simulink library "dspbuff3"  (Simulink 5.0)
libraries: dspbuff3 x1
settings Model: RequirementInfo=9  CovMetricSettings=d  Creator=szlotkin  LastModifiedBy=mkhan  TargetHWChar=2  TargetHWWordLengths=8,16,32,32

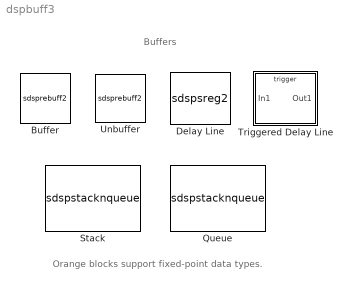
== system dspbuff3 ==
  note: Buffers
  note: Orange blocks support fixed-point data types.
  Buffer : S-Function  FunctionName=sdsprebuff2  Parameters=N,V,ic  mask(Buffer){N=64, V=0, ic=0}
      mask prompts: N "Output buffer size (per channel):"; V "Buffer overlap:"; ic "Initial conditions:"
      mask help:
      | Convert scalar samples to a frame output at a lower sample rate.  You can also convert a frame to a smaller or larger size with optional overlap.
      | For calculation of sample delay, see the rebuffer_delay function.
      mask init:
      | [x,y] = dspblkbuff('icon');
      settings: CopyFcn=dspfixptcopycallback
      mask Help: web(dspbhelp);
      mask Display: plot(x,y)
  Delay Line : S-Function  FunctionName=sdspsreg2  Parameters=siz,ic,directfeed  mask(Delay Line){siz=64, ic=0, directfeed=off}
      mask prompts: siz "Delay line size:"; ic "Initial conditions:"; directfeed "Allow directfeedthrough"
      mask help: Shift out delay line contents and store input data into start of delay line.
      settings: CopyFcn=dspfixptcopycallback
      mask Help: web(dspbhelp);
      mask Display: disp('Delay\nLine');
  Queue : S-Function  FunctionName=sdspstacknqueue  Parameters=trigger,depth,overflow,pes,eso,fso,nso,clr,clrOutport,1  mask(Queue){depth=8, trigger=Rising edge, overflow=Dynamic reallocation, pes=Warning, eso=off, fso=off, nso=off, clr=off, clrOutport=off}
      mask prompts: depth "Register size:"; trigger "Trigger type:"; overflow "Push onto full register:"; pes "Pop empty register:"; eso "Empty register output"; fso "Full register output"; nso "Output number of register entries"; clr "Clear input"; clrOutport "Clear output port on reset"
      mask help: Implements a queue, or "First In, First Out" (FIFO) register.
      mask init:
      | [si,so] = dspblkstack('icon', clr,eso,fso,nso);
      settings: CopyFcn=dspfixptcopycallback
      mask Help: web(dspbhelp);
      mask StyleString: edit,popup(Rising edge|Falling edge|Either edge|Non-zero sample),popup(Dynamic reallocation|Ignore|Warning|Error),popup(Ignore|Warning|Error),checkbox,checkbox,checkbox,checkbox,checkbox
      mask Display:
      | disp('Queue');
      | 
      | port_label('input',si(1).port, si(1).txt);
      | port_label('input',si(2).port, si(2).txt);
      | port_label('input',si(3).port, si(3).txt);
      | port_label('input',si(4).port, si(4).txt);
      | 
      | port_label('output',so(1).port, so(1).txt);
      | port_label('output',so(2).port, so(2).txt);
      | port_label('output',so(3).port, so(3).txt);
      | port_label('output',so(4).port, so(4).txt);
  Stack : S-Function  FunctionName=sdspstacknqueue  Parameters=trigger,depth,overflow,pes,eso,fso,nso,clr,clrOutport,0  mask(Stack){depth=8, trigger=Rising edge, overflow=Dynamic reallocation, pes=Warning, eso=off, fso=off, nso=off, clr=off, clrOutport=off}
      mask prompts: depth "Stack depth:"; trigger "Trigger type:"; overflow "Push full stack:"; pes "Pop empty stack:"; eso "Empty stack output"; fso "Full stack output"; nso "Output number of stack entries"; clr "Clear input"; clrOutport "Clear output port on reset"
      mask help: Implements a stack, or "Last In, First Out" (LIFO) register.
      mask init:
      | [si,so] = dspblkstack('icon', clr,eso,fso,nso);
      settings: CopyFcn=dspfixptcopycallback
      mask Help: web(dspbhelp);
      mask StyleString: edit,popup(Rising edge|Falling edge|Either edge|Non-zero sample),popup(Dynamic reallocation|Ignore|Warning|Error),popup(Ignore|Warning|Error),checkbox,checkbox,checkbox,checkbox,checkbox
      mask Display:
      | disp('Stack');
      | 
      | port_label('input',si(1).port, si(1).txt);
      | port_label('input',si(2).port, si(2).txt);
      | port_label('input',si(3).port, si(3).txt);
      | port_label('input',si(4).port, si(4).txt);
      | 
      | port_label('output',so(1).port, so(1).txt);
      | port_label('output',so(2).port, so(2).txt);
      | port_label('output',so(3).port, so(3).txt);
      | port_label('output',so(4).port, so(4).txt);
  Triggered Delay Line : Subsystem  TreatAsAtomicUnit=on  mask(Triggered Delay Line){trig=Rising edge, siz=64, ic=0}
      mask prompts: trig "Trigger type:"; siz "Delay line size:"; ic "Initial conditions:"
      mask help: Shift out delay line contents and store input data into start of delay line when trigger event occurs.
      mask init:
      | switch trig
      | case 1, s='rising';
      | case 2, s='falling';
      | case 3, s='either';
      | end
      | set_param([gcb '/Trigger'],'triggertype',s);
      settings: CopyFcn=dspfixptcopycallback
      mask Help: web(dspbhelp);
      mask StyleString: popup(Rising edge|Falling edge|Either edge),edit,edit
      mask Display: disp('Delay\nLine');
  Unbuffer : S-Function  FunctionName=sdsprebuff2  Parameters=1,0,ic  mask(Unbuffer){ic=0}
      mask prompts: ic "Initial conditions:"
      mask help: Convert a frame to scalar samples output at a higher sample rate.
      settings: CopyFcn=dspfixptcopycallback
      mask Help: web(dspbhelp);
      mask Display: plot(0,0,100,100,[62 68 68 72 68 68],[24 24 26 24 22 24],[36 36 56 49 56 49],[32 24 24 16 24 32],[20 52 52 20 20],[88 88 36 36 88],[28 44],[80 80],[28 44],[72 72],[28 44],[64 64],[28 44],[56 56],[28 44],[48 48],[72 76 76 80 76 76],[24 24 26 24 22 24],[80 84 84 88 84 84],[24 24 26 24 22 24],[],[],[],[],[88 88 92],[24 24 24])

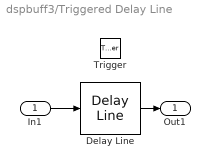
== system dspbuff3/Triggered Delay Line ==
  In1 : Inport
  Trigger : TriggerPort  ZeroCross=off
  Delay Line : dspbuff3/Delay Line  siz=siz  ic=ic  directfeed=off
  Out1 : Outport  InitialOutput=ic
  wires:
  Delay Line/1 -> Out1/1
  In1/1 -> Delay Line/1
